simulink model "Sample150"  (Simulink 6.3)
settings: Solver=ode45  StartTime=0.0  StopTime=10.0  RelTol=1e-3
undefined symbols (not defined in the file): get
libraries: commdigbbndfm2 x3, dspsnks4 x2, commblkcod2 x2, dspbuff3 x2, simulink x2, commrandsrc2 x1, commchan3 x1, commsink2 x1, commdigbbndcpm2 x1
settings Model: LastModifiedBy=Administrator

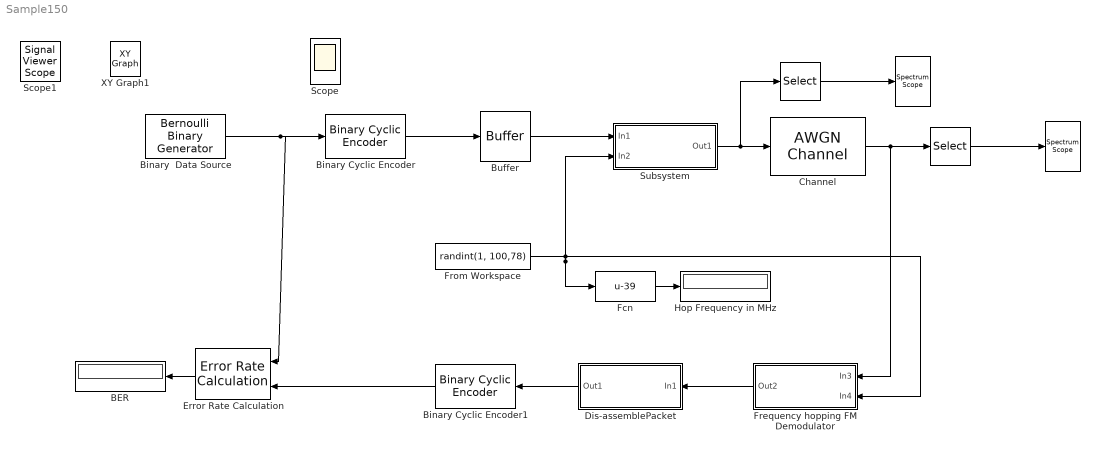
== system Sample150 ==
  " " : Selector  InputType=Matrix  Elements=[1 3]  Rows=1:512  InputPortWidth=3
  "  " : dspsnks4/Spectrum Scope  DialogController=dspdialog.SpectrumScope  DialogControllerArgs=DataTag0  ScopeProperties=on  Domain=Frequency  HorizSpan=1  UseBuffer=off  BufferSize=128  Overlap=64  inpFftLenInherit=off  FFTlength=128  numAvg=2  DisplayProperties=off  AxisGrid=off  Memory=off  FrameNumber=on  AxisLegend=off  AxisZoom=off  OpenScopeAtSimStart=on  OpenScopeImmediately=off  FigPos=get(0,'defaultfigureposition')  AxisProperties=off  XUnits=Hertz  XRange=[0...Fs/2]  InheritXIncr=on  XIncr=1.0  XLabel=Samples  YUnits=dB  YLabel=Magnitude-squared, dB  LineProperties=off  wintypeSpecScope=Hann  RsSpecScope=50  betaSpecScope=5  winsampSpecScope=Periodic
      settings: YMin=-10  YMax=10
  "    " : dspsnks4/Spectrum Scope  DialogController=dspdialog.SpectrumScope  DialogControllerArgs=DataTag1  ScopeProperties=on  Domain=Frequency  HorizSpan=1  UseBuffer=off  BufferSize=128  Overlap=64  inpFftLenInherit=off  FFTlength=128  numAvg=2  DisplayProperties=off  AxisGrid=on  Memory=off  FrameNumber=on  AxisLegend=off  AxisZoom=off  OpenScopeAtSimStart=on  OpenScopeImmediately=off  FigPos=get(0,'defaultfigureposition')  AxisProperties=off  XUnits=Hertz  XRange=[0...Fs/2]  InheritXIncr=on  XIncr=1.0  XLabel=Samples  YUnits=dB  YLabel=Magnitude-squared, dB  LineProperties=off  wintypeSpecScope=Hann  RsSpecScope=50  betaSpecScope=5  winsampSpecScope=Periodic
      settings: YMin=-10  YMax=10
  "     " : Selector  InputType=Matrix  Elements=[1 3]  Rows=1:512  InputPortWidth=3
  BER : Display
  Binary Cyclic Encoder : commblkcod2/Binary Cyclic Encoder  n=15  p=[1 1 0 1 0 1]
  Binary Cyclic Encoder1 : commblkcod2/Binary Cyclic Encoder  Orientation=left  n=15  p=[1 1 0 1 0 1]
  Binary  Data Source : commrandsrc2/Bernoulli Binary Generator  P=[.5]  seed=[12345]  Ts=1.5e-6  frameBased=on  sampPerFrame=10  orient=off  outDataType=double
  Buffer : dspbuff3/Buffer  N=625  V=0  ic=0
  Channel : commchan3/AWGN Channel  seed=1  noiseMode="Signal to noise ratio  (Eb/No)"  EbNodB=20  EsNodB=10  SNRdB=10  bitsPerSym=1  Ps=1  Tsym=1e-6  variance=1
  Dis-assemblePacket : Subsystem  Orientation=left
  Error Rate Calculation : commsink2/Error Rate Calculation  Orientation=left  N=850  st_delay=0  cp_mode=Entire frame  subframe=[]  PMode=Port  WsName=ErrorVec  RsMode2=off  stop=off  numErr=100  maxBits=1e6
  Fcn : Fcn  Expr=u-39
  Frequency hopping FM Demodulator : Subsystem  Orientation=left
  From Workspace : FromWorkspace  VariableName=randint(1, 100,78)  SampleTime=1/1600
  Hop Frequency in MHz : Display
  Scope : Scope
  Subsystem : Subsystem
  Scope1 : SignalViewerScope  IOType=viewer  RefreshTime=0.035000
  XY Graph1 : simulink/Sinks/XY Graph  IOType=viewer  xmin=-1  xmax=1  ymin=-1  ymax=1  st=-1
  wires:
  Binary Cyclic Encoder/1 -> Buffer/1
  Buffer/1 -> Subsystem/1(In1)
  From Workspace/1 -> Subsystem/2(In2), Frequency hopping FM Demodulator/2(In4), Fcn/1
  Subsystem/1(Out1) -> " "/1, Channel/1
  " "/1 -> "  "/1
  "     "/1 -> "    "/1
  Channel/1 -> "     "/1, Frequency hopping FM Demodulator/1(In3)
  Fcn/1 -> Hop Frequency in MHz/1
  Frequency hopping FM Demodulator/1(Out2) -> Dis-assemblePacket/1(In1)
  Dis-assemblePacket/1(Out1) -> Binary Cyclic Encoder1/1
  Binary Cyclic Encoder1/1 -> Error Rate Calculation/2
  Error Rate Calculation/1 -> BER/1
  Binary  Data Source/1 -> Binary Cyclic Encoder/1, Error Rate Calculation/1

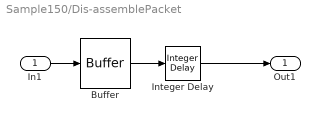
== system Sample150/Dis-assemblePacket ==
  In1 : Inport
  Buffer : dspbuff3/Buffer  N=15  V=0  ic=0
  Integer Delay : simulink/Discrete/Integer Delay  vinit=0.0  samptime=-1  NumDelays=10
  Out1 : Outport
  wires:
  In1/1 -> Buffer/1
  Buffer/1 -> Integer Delay/1
  Integer Delay/1 -> Out1/1

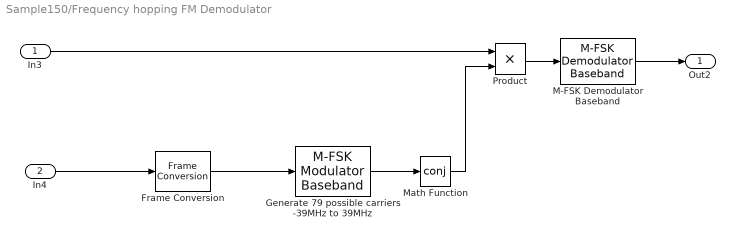
== system Sample150/Frequency hopping FM Demodulator ==
  In3 : Inport
  In4 : Inport  Port=2
  Frame Conversion : FrameConversion
  Generate 79 possible carriers -39MHz to 39MHz : commdigbbndfm2/M-FSK Modulator Baseband  M=19  InType=Integer  Enc=Binary  freqSep=1e6  phaseType=Continuous  numSamp=6.25e4  outDataType=double
  M-FSK Demodulator Baseband : commdigbbndfm2/M-FSK Demodulator Baseband  M=2  OutType=Integer  Dec=Binary  freqSep=10  numSamp=100  outDataType=double
  Math Function : Math  Operator=conj  SaturateOnIntegerOverflow=on
  Product : Product  RndMeth=Zero
  Out2 : Outport
  wires:
  In3/1 -> Product/1
  Frame Conversion/1 -> Generate 79 possible carriers -39MHz to 39MHz/1
  In4/1 -> Frame Conversion/1
  Generate 79 possible carriers -39MHz to 39MHz/1 -> Math Function/1
  Math Function/1 -> Product/2
  Product/1 -> M-FSK Demodulator Baseband/1
  M-FSK Demodulator Baseband/1 -> Out2/1

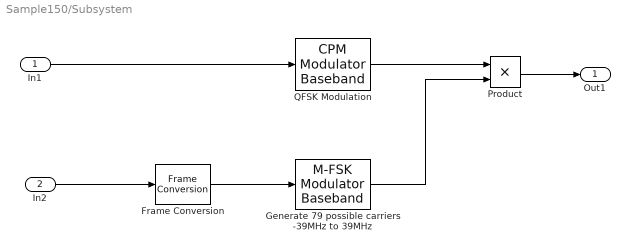
== system Sample150/Subsystem ==
  In1 : Inport
  In2 : Inport  Port=2
  Frame Conversion : FrameConversion
  Generate 79 possible carriers -39MHz to 39MHz : commdigbbndfm2/M-FSK Modulator Baseband  M=79  InType=Integer  Enc=Binary  freqSep=1e6  phaseType=Continuous  numSamp=6.25e4  outDataType=double
  Product : Product  RndMeth=Zero
  QFSK Modulation : commdigbbndcpm2/CPM Modulator Baseband  Mnum=2  inputType=Bit  mappingType=Binary  modIdx=0.3  pulseShape=Gaussian  BT=0.5  mainLobePulseLength=1  rollOff=0.2  pulseLength=1  preHistory=1  phaseOffset=0  samplesPerSymbol=8  outDataType=double
  Out1 : Outport
  wires:
  Product/1 -> Out1/1
  Generate 79 possible carriers -39MHz to 39MHz/1 -> Product/2
  QFSK Modulation/1 -> Product/1
  In1/1 -> QFSK Modulation/1
  Frame Conversion/1 -> Generate 79 possible carriers -39MHz to 39MHz/1
  In2/1 -> Frame Conversion/1
